simulink model "dot_animation"  (Simulink 6.1)
settings: Solver=ode45  StartTime=0.0  StopTime=10000  MaxStep=0.1  RelTol=1e-3
undefined symbols (not defined in the file or in its folder): ansim
settings Model: LastModifiedBy=End User
settings DebuggingCC: SolverPrmCheckMsg=warning

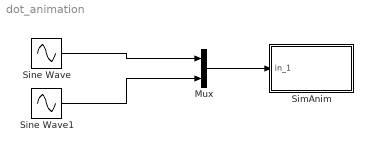
== system dot_animation ==
  Mux : Mux  Inputs=2
  SimAnim : Subsystem
      settings: NameChangeFcn=ansim([],[],[],'NameChange');  OpenFcn=ansimini #Initialize
      mask Type: Simulation Animation
      mask Help: dot_animation.mat
      mask Display: disp('Simulation\nAnimation')
  Sine Wave : Sin  Frequency=10  SampleTime=0
  Sine Wave1 : Sin  Frequency=30  Phase=90  SampleTime=0
  wires:
  Sine Wave/1 -> Mux/1
  Sine Wave1/1 -> Mux/2
  Mux/1 -> SimAnim/1(in_1)

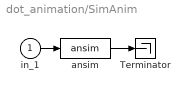
== system dot_animation/SimAnim ==
  in_1 : Inport  Port=1  LatchInput=off
  Terminator : Terminator
  ansim : S-Function  LoadFcn=ansim([],[],[],'LoadBlock');  StartFcn=ansim([],[],[],'Start');  StopFcn=ansim([],[],[],'Stop');  FunctionName=ansim  Parameters=1
      settings: CopyFcn=ansim([],[],[],'CopyBlock');  DeleteFcn=ansim([],[],[],'DeleteBlock');
  wires:
  in_1/1 -> ansim/1
  ansim/1 -> Terminator/1
